simulink model "automata_learning"  (R2018a)
settings: Solver=FixedStepAuto  StartTime=0.0  StopTime=T  FixedStep=Ts  RelTol=1e-3
libraries: simulink x1
settings Model: Creator=xiaodong  LastModifiedBy=xiaodong

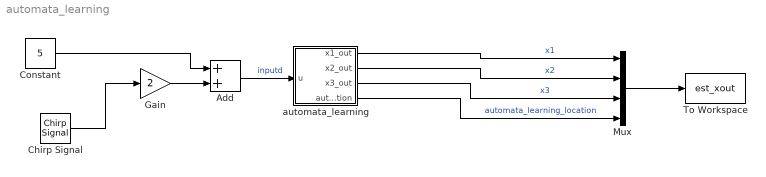
== system automata_learning ==
  Add : Sum
  Chirp Signal : simulink/Sources/Chirp Signal  f1=0.001  T=100  f2=0.01
  Constant : Constant  Value=5
  Gain : Gain  Gain=2
  Mux : Mux
  To Workspace : ToWorkspace  VariableName=est_xout  SampleTime=-1
  automata_learning : Stateflow chart  TreatAsAtomicUnit=on
  wires:
  automata_learning/1(x1_out) -> Mux/1  "x1"
  automata_learning/2(x2_out) -> Mux/2  "x2"
  automata_learning/3(x3_out) -> Mux/3  "x3"
  automata_learning/4(automata_learning_location) -> Mux/4  "automata_learning_location"
  Constant/1 -> Add/1
  Chirp Signal/1 -> Gain/1
  Add/1 -> automata_learning/1(u)  "inputd"
  Gain/1 -> Add/2
  Mux/1 -> To Workspace/1

== stateflow chart automata_learning/automata_learning ==
  settings: updateMethod=CONTINUOUS
  state loc2
    du:
    x1_dot = 0.02983110936037292 * x2 - 0.10009188445428663 * x1 + 0.04001825733348596 * x3 + 0.003670540986639992 +0.0300712836076816*u;
    x2_dot = 0.029938832714890395 * x1 - 0.1001124537197029 * x2 + 0.05001216143091369 * x3 + 0.0024436763565773845+0.0200474586573245*u;
    x3_dot = 0.03984668427960969 * x1 + 0.04971814957445986 * x2 - 0.13996957396375365 * x3 + 1.1061260487040272+0.0501189655741881*u;
    x1_out=x1;
    x2_out=x2;
    x3_out=x3;
    automata_learning_location =2;
  state loc3
    du:
    x1_dot = 0.09343506368327326 * x3 - 0.0768821962135462 * x2 - 0.05341383530003441 * x1 + 0.9197662889964704+0.0230617736319312*u;
    x2_dot = 0.02988717956088749 * x1 - 0.09993327360325566 * x2 + 0.05004681230775532 * x3 + 0.000007468157300252742+0.0200346673215340*u;
    x3_dot = 0.03971729915588185 * x1 + 0.05016703087642327 * x2 - 0.13988245556402035 * x3 + 0.00001723801284819748+0.0500868559595906*u;
    x1_out=x1;
    x2_out=x2;
    x3_out=x3;
    automata_learning_location =3;
  state loc5
    du:
    x1_dot = 0.02991490722291701 * x2 - 0.10025706683632052 * x1 + 0.03973912049514183 * x3 + 0.006193401834465817+0.0303018362806778*u;
    x2_dot = 0.029828865079934985 * x1 - 0.10005666806500813 * x2 + 0.04982632963992728 * x3 + 0.004123277207327192+0.0202009476997724*u;
    x3_dot = 0.039570999050056344 * x1 + 0.04985800978124644 * x2 - 0.1404354445003264 * x3 + 0.010336345839021988+0.0505037468555066*u;
    x1_out=x1;
    x2_out=x2;
    x3_out=x3;
    automata_learning_location =5;
  state loc6
    du:
    x1_dot = 0.02991490722291701 * x2 - 0.10025706683632052 * x1 + 0.03973912049514183 * x3 + 0.006193401834465817+0.0303018362806778*u;
    x2_dot = 0.029828865079934985 * x1 - 0.10005666806500813 * x2 + 0.04982632963992728 * x3 + 0.004123277207327192+0.0202009476997724*u;
    x3_dot = 0.039570999050056344 * x1 + 0.04985800978124644 * x2 - 0.1404354445003264 * x3 + 0.010336345839021988+0.0505037468555066*u;
    x1_out=x1;
    x2_out=x2;
    x3_out=x3;
    automata_learning_location =6;
  state loc4
    du:
    x1_dot = 0.02991490722291701 * x2 - 0.10025706683632052 * x1 + 0.03973912049514183 * x3 + 0.006193401834465817+0.0303018362806778*u;
    x2_dot = 0.029828865079934985 * x1 - 0.10005666806500813 * x2 + 0.04982632963992728 * x3 + 0.004123277207327192+0.0202009476997724*u;
    x3_dot = 0.039570999050056344 * x1 + 0.04985800978124644 * x2 - 0.1404354445003264 * x3 + 0.010336345839021988+0.0505037468555066*u;
    x1_out=x1;
    x2_out=x2;
    x3_out=x3;
    automata_learning_location =4;
  state loc1
    du:
    x1_dot = 0.030158665636008664 * x2 - 0.09947919446267406 * x1 + 0.039360045440275826 * x3 - 0.002674285621807826+0.0301018616366555*u;
    x2_dot = 0.010812596275485475 * x1 - 0.08157654470778652 * x2 + 0.0186715357014009 * x3 + 1.1037585892590869+0.0235172515927914*u;
    x3_dot = 0.04086923046463653 * x1 + 0.050264821390783254 * x2 - 0.14106810223120192 * x3 - 0.004463351981769392+0.0501700056271048*u;
    x1_out=x1;
    x2_out=x2;
    x3_out=x3;
    automata_learning_location =1;
  loc6 -> loc3 : [0.0005937 * x3 - 0.001096 * x2 - 0.04963 * x1 + 1.0 > 0.0]
  loc4 -> loc1 : [0.0007212 * x3 - 0.05266 * x2 - 0.0007331 * x1 + 1.0 > 0.0]
  loc3 -> loc1 [order 1] : [0.32914761011488736 * x2 - 0.330816243929803 * x1 + 0.0016025840094222588 * x3 + 1.0 < 0.0 && 0.000747881469045808 * x1 - 0.06493177253923932 * x2 + 0.0015819446342675292 * x3 + 1.0 > 0.0]
  loc1 -> loc2 [order 1] : [0.00024371532852418554 * x1 - 0.47941399145020114 * x2 + 0.47701453661193227 * x3 + 1.0 < 0.0 && 0.00041738168303329104 * x2 - 0.0013751061795019837 * x1 - 0.06585387725635883 * x3 + 1.0 > 0.0]
  loc2 -> loc3 [order 1] : [0.4886526159425557 * x1 + 0.001216676004972328 * x2 - 0.4903256963525564 * x3 + 1.0 < 0.0 && 0.0003015183846786229 * x2 - 0.06271767129419459 * x1 - 0.00009015019658331624 * x3 + 1.0 > 0.0]
  (default) -> loc1 : {x1 = x_init(1);
      | x2 = x_init(2);
      | x3 = x_init(3);}
  loc5 -> loc2 : [0.0006491 * x1 + 0.0005503 * x2 - 0.05381 * x3 + 1.0 > 0.0]
  loc2 -> loc5 [order 2] : [0.0002148 * x2 - 0.00004384 * x1 - 0.04556 * x3 + 1.0 < 0.0]
  loc3 -> loc6 [order 2] : [0.0004999 * x3 - 0.0007582 * x2 - 0.04737 * x1 + 1.0 < 0.0]
  loc1 -> loc4 [order 2] : [0.0007874 * x3 - 0.04794 * x2 - 0.0003544 * x1 + 1.0 < 0.0]
  data: x1_out output; x1 local; x2_out output; x2 local; x3_out output; x3 local; automata_learning_location output; u input; x_init constant double size=3 =x_init
  data x1 settings: updateMethod=SF_CONTINUOUS_TIME_DATA
  data x2 settings: updateMethod=SF_CONTINUOUS_TIME_DATA
  data x3 settings: updateMethod=SF_CONTINUOUS_TIME_DATA
